simulink model "linealizada1"  (Simulink 7.3)
settings: Solver=ode45  StartTime=0.0  StopTime=15000  MaxStep=0.03  MinStep=0.01  RelTol=1e-3
libraries: dspsigops x7
settings Model: Creator=root  LastModifiedBy=Daniel
settings SolverCC: InitialStep=0.01
settings DebuggingCC: FcnCallInpInsideContextMsg=Enable All  StrictBusMsg=ErrorLevel1
settings GRTTargetCC: CombineOutputUpdateFcns=on

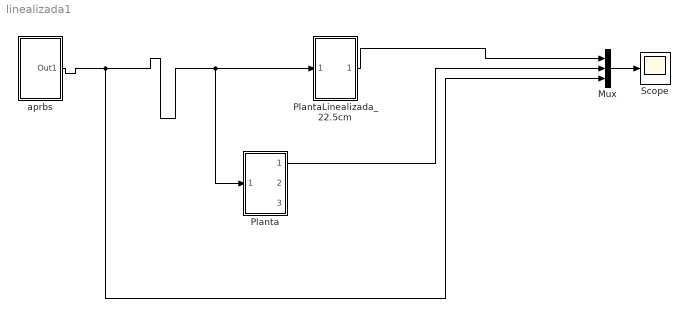
== system linealizada1 ==
  Mux : Mux  Inputs=3
  Planta : Subsystem
  PlantaLinealizada_22.5cm : Subsystem
  Scope : Scope
      settings: DataFormat=Array
  aprbs : Subsystem
  wires:
  Mux/1 -> Scope/1
  aprbs/1(Out1) -> Mux/3, PlantaLinealizada_22.5cm/1(In1), Planta/1(In1)
  PlantaLinealizada_22.5cm/1(Out1) -> Mux/1
  Planta/1(Out1) -> Mux/2

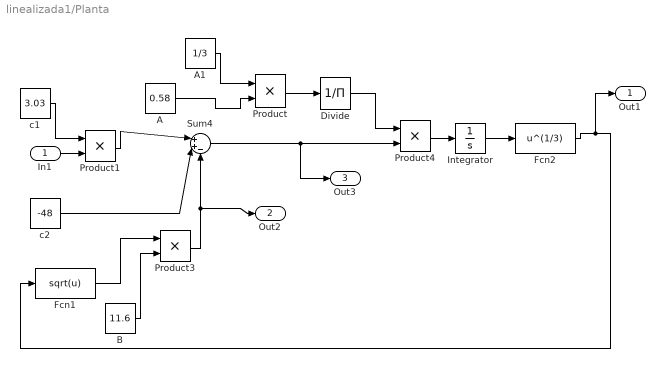
== system linealizada1/Planta ==
  In1 : Inport
  A : Constant  Value=0.58
  A1 : Constant  Value=1/3
  B : Constant  Value=11.6
  Divide : Product  Inputs=/
  Fcn1 : Fcn  Expr=sqrt(u)  SampleTime=0.1
  Fcn2 : Fcn  Expr=u^(1/3)  SampleTime=0.1
  Integrator : Integrator  InitialCondition=22.5^3  LowerSaturationLimit=0.1
  Product : Product  Inputs=**  RndMeth=Zero
  Product1 : Product  SampleTime=0.1  RndMeth=Zero
  Product3 : Product  SampleTime=0.1  RndMeth=Zero
  Product4 : Product  SampleTime=0.1  RndMeth=Zero
  Sum4 : Sum  Inputs=|++-
  c1 : Constant  Value=3.03
  c2 : Constant  Value=-48
  Out1 : Outport
  Out2 : Outport  Port=2
  Out3 : Outport  Port=3
  wires:
  c1/1 -> Product1/1
  Product1/1 -> Sum4/1
  c2/1 -> Sum4/2
  Fcn1/1 -> Product3/1
  B/1 -> Product3/2
  Product3/1 -> Sum4/3, Out2/1
  Sum4/1 -> Product4/2, Out3/1
  Divide/1 -> Product4/1
  Product/1 -> Divide/1
  Product4/1 -> Integrator/1
  In1/1 -> Product1/2
  A/1 -> Product/2
  A1/1 -> Product/1
  Integrator/1 -> Fcn2/1
  Fcn2/1 -> Fcn1/1, Out1/1

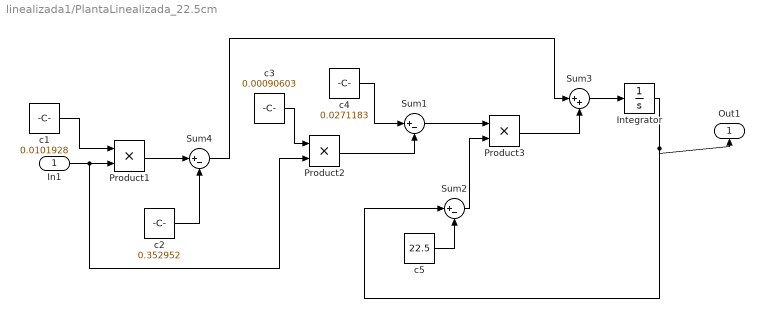
== system linealizada1/PlantaLinealizada_22.5cm ==
  In1 : Inport
  Integrator : Integrator  InitialCondition=10  UpperSaturationLimit=70  LowerSaturationLimit=0.1
  Product1 : Product  SampleTime=0.1  RndMeth=Zero
  Product2 : Product  SampleTime=0.1  RndMeth=Zero
  Product3 : Product  SampleTime=0.1  RndMeth=Zero
  Sum1 : Sum  Inputs=|+-
  Sum2 : Sum  Inputs=|+-
  Sum3 : Sum  Inputs=|++
  Sum4 : Sum  Inputs=|+-
  c1 : Constant  Value=0.0101928
  c2 : Constant  Value=0.352952
  c3 : Constant  Value=0.00090603
  c4 : Constant  Value=0.0271183
  c5 : Constant  Value=22.5
  Out1 : Outport
  wires:
  c1/1 -> Product1/1
  In1/1 -> Product1/2, Product2/2
  Product1/1 -> Sum4/1
  c2/1 -> Sum4/2
  c3/1 -> Product2/1
  Product2/1 -> Sum1/2
  c4/1 -> Sum1/1
  c5/1 -> Sum2/2
  Sum2/1 -> Product3/2
  Sum1/1 -> Product3/1
  Product3/1 -> Sum3/2
  Sum4/1 -> Sum3/1
  Sum3/1 -> Integrator/1
  Integrator/1 -> Sum2/1, Out1/1

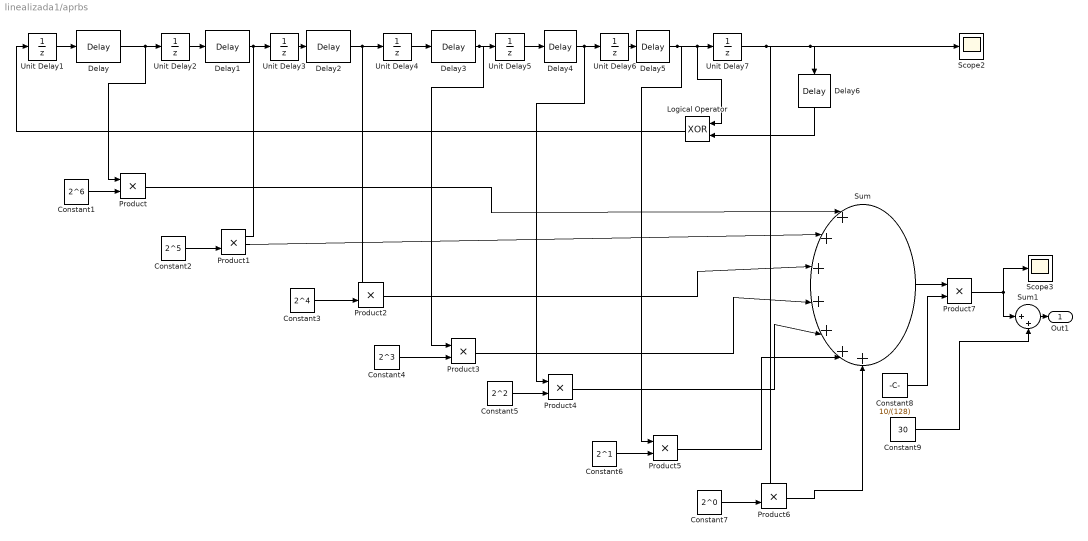
== system linealizada1/aprbs ==
  Constant1 : Constant  Value=2^6
  Constant2 : Constant  Value=2^5
  Constant3 : Constant  Value=2^4
  Constant4 : Constant  Value=2^3
  Constant5 : Constant  Value=2^2
  Constant6 : Constant  Value=2^1
  Constant7 : Constant  Value=2^0
  Constant8 : Constant  Value=10/(128)
  Constant9 : Constant  Value=30
  Delay{,1..6} (7 alike) : dspsigops/Delay  dly_unit=Samples  delay=1200  ic_detail=off  dif_ic_for_ch=off  dif_ic_for_dly=off  ic=1  reset_popup=None
  Logical Operator : Logic  Operator=XOR  AllPortsSameDT=off  OutDataTypeMode=boolean  OutDataTypeStr=boolean
  Product{,1..6} (7 alike) : Product  RndMeth=Zero
  Product7 : Product  SampleTime=0.1  RndMeth=Zero
  Scope2 : Scope
      settings: SaveName=ScopeData2  DataFormat=Array
  Scope3 : Scope
      settings: SaveName=ScopeData3
  Sum : Sum  Inputs=|+++++++  SampleTime=0.1
  Sum1 : Sum  Inputs=|++  SampleTime=0.1
  Unit Delay{1..7} (7 alike) : UnitDelay  X0=1  SampleTime=0.1
  Out1 : Outport
  wires:
  Unit Delay2/1 -> Delay1/1
  Unit Delay3/1 -> Delay2/1
  Unit Delay5/1 -> Delay4/1
  Logical Operator/1 -> Unit Delay1/1
  Unit Delay6/1 -> Delay5/1
  Unit Delay7/1 -> Product6/1, Scope2/1, Delay6/1
  Product/1 -> Sum/1
  Product1/1 -> Sum/2
  Product2/1 -> Sum/3
  Product3/1 -> Sum/4
  Product4/1 -> Sum/5
  Product5/1 -> Sum/6
  Product6/1 -> Sum/7
  Constant1/1 -> Product/2
  Constant2/1 -> Product1/2
  Constant3/1 -> Product2/2
  Constant4/1 -> Product3/2
  Constant7/1 -> Product6/2
  Constant6/1 -> Product5/2
  Constant5/1 -> Product4/2
  Sum/1 -> Product7/1
  Unit Delay1/1 -> Delay/1
  Delay/1 -> Unit Delay2/1, Product/1
  Delay1/1 -> Unit Delay3/1, Product1/1
  Delay2/1 -> Unit Delay4/1, Product2/1
  Unit Delay4/1 -> Delay3/1
  Delay3/1 -> Unit Delay5/1, Product3/1
  Delay4/1 -> Unit Delay6/1, Product4/1
  Delay5/1 -> Unit Delay7/1, Logical Operator/1, Product5/1
  Delay6/1 -> Logical Operator/2
  Constant9/1 -> Sum1/2
  Constant8/1 -> Product7/2
  Product7/1 -> Sum1/1, Scope3/1
  Sum1/1 -> Out1/1
